simulink model "Asyn_Demodulator"  (R2014b)
settings: Solver=ode3  StartTime=0.0  StopTime=1  FixedStep=1/5000000  RelTol=1e-3
undefined symbols (not defined in the file or in its folder): dfilt, fdesignblkfcn, gcbh
libraries: dsparch4 x1
settings Model: Creator=Eitima  LastModifiedBy=Eitima
settings DataIOCC: ExternalInput=[t, SigTime]  LimitDataPoints=off  LoadExternalInput=on  TimeSaveName=tOut  OutputSaveName=SigTimeOut

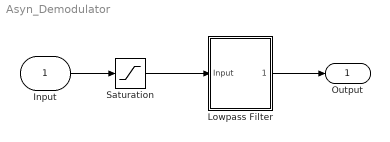
== system Asyn_Demodulator ==
  Input : Inport
  Lowpass Filter : Subsystem
  Saturation : Saturate  UpperLimit=inf  LowerLimit=0
  Output : Outport
  wires:
  Lowpass Filter/1(Output) -> Output/1
  Saturation/1 -> Lowpass Filter/1(Input)
  Input/1 -> Saturation/1

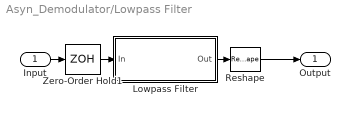
== system Asyn_Demodulator/Lowpass Filter ==
  Input : Inport
  Lowpass Filter : Subsystem  DialogController=fdesignblkfcn  InitFcn=fdesignblkfcn(gcbh, {'InitFcn'});  mask(Lowpass Filter){}
      mask help: Design a lowpass filter
      settings: CopyFcn=fdesignblkfcn(gcbh, {'CopyFcn'});
      mask Help: helpview(mapfilelocation('dsp'), 'dsplowpassfilter');
      mask Display: disp('Lowpass')
  Reshape : Reshape
  Zero-Order Hold1 : ZeroOrderHold  SampleTime=-1
  Output : Outport
  wires:
  Zero-Order Hold1/1 -> Lowpass Filter/1(In)
  Input/1 -> Zero-Order Hold1/1
  Lowpass Filter/1(Out) -> Reshape/1
  Reshape/1 -> Output/1

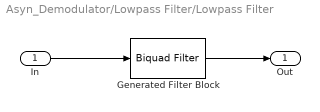
== system Asyn_Demodulator/Lowpass Filter/Lowpass Filter ==
  In : Inport
  Generated Filter Block : dsparch4/Biquad Filter  Tag=BlockMethodSubSystem  IIRFiltStruct=Direct form II  CoeffSource=Specify via dialog  BiQuadCoeffs=[1.1139495474470017e-05 2.2278990948940034e-05 1.1139495474470017e-05 1 -1.9975472496899784 0.99760587630988296;1.708449290031526e-05 3.4168985800630521e-05 1.708449290031526e-05 1 -1.99387457640288 0.99393309523238282;2.1150286544110928e-05 4.2300573088221855e-05 2.1150286544110928e-05 1 -1.9905941002634866 0.99065252281330018;2.3741131754506419e-05 4.7482263509012838e-05 2.3741131754506419e-05 1 -1.9879072271736171 0.9879655708655779;2.2148688266151217e-05 4.4297376532302434e-05 2.2148688266151217e-05 1 -1.9859774513096744 0.98603573836405833;1.4562706238119281e-05 2.9125412476238562e-05 1.4562706238119281e-05 1 -1.9849213847063547 0.98497964076591971;1.4567049256231092e-05 2.9134098512462184e-05 1.4567049256231092e-05 1 -1.9847430291087753 0.98480127993372768;1.457808673549499e-05 2.915617347098998e-05 1.457808673549499e-05 1 -1.9853349366021702 0.98539320479919512;1.4595153426943952e-05 2.9190306853887904e-05 1.4595153426943952e-05 1 -1.986839228435767 0.98689754078270897;1.4617214727563608e-05 2.9234429455127217e-05 1.4617214727563608e-05 1 -1.9891652381977778 0.98922361881148557;1.4642922502972056e-05 2.9285845005944111e-05 1.4642922502972056e-05 1 -1.9921719604380583 0.99223042929696859;8.6714112246987757e-06 1.7342822449397551e-05 8.6714112246987757e-06 1 -1.995675658652956 0.99573423034296782;6.3986527910792821e-06 1.2797305582158564e-05 6.3986527910792821e-06 1 -1.9994601364673172 0.99951881922911578;1.3142520276408514e-05 2.6285040552817028e-05 1.3142520276408514e-05 1 -1.9966044420030755 0.99666304095223146;1.8418289343954956e-05 3.6836578687909913e-05 1.8418289343954956e-05 1 -1.9930092733310447 0.99306776676450537;2.2982277427308612e-05 4.5964554854617224e-05 2.2982277427308612e-05 1 -1.9898596189140614 0.98991801990735939;2.6110938013399351e-05 5.2221876026798703e-05 2.6110938013399351e-05 1 -1.9873483912460574 0.98740671853657336;1.7614429604367743e-05 3.5228859208735487e-05 1.7614429604367743e-05 1 -1.9856280998827738 0.98568637668393688;1.4565318613601885e-05 2.9130637227203771e-05 1.4565318613601885e-05 1 -1.9848025557236171 0.98486080829563394;1.4574729484739814e-05 2.9149458969479628e-05 1.4574729484739814e-05 1 -1.9850990682844676 0.98515732955892188;1.4590372236056304e-05 2.9180744472112607e-05 1.4590372236056304e-05 1 -1.9863816706239454 0.98643996954188451;1.4611300168831942e-05 2.9222600337663884e-05 1.4611300168831942e-05 1 -1.9885136123818619 0.98857197387080598;1.4636237197718225e-05 2.9272474395436451e-05 1.4636237197718225e-05 1 -1.9913658685524318 0.99142431375310713;1.4663493412127055e-05 2.9326986824254111e-05 1.4663493412127055e-05 1 -1.9947645221736521 0.99482306712244295;0.25000264423165819 0.50000528846331638 0.25000264423165819 1 -1.9985003940838757 0.99855904867790413]  a0Flag=Warning  IC=0  ICnum=0  ICden=0  InputProcessing=Columns as channels (frame based)  denAccumFracLength=30  denProdOutputFracLength=30  secondMemoryFracLength=15  roundingMode=Floor  overflowMode=off  ScaleValues=[1.8320818000818615e-05;1;1;1;1;1;1;1;1;1;1;1;1;1;1;1;1;1;1;1;1;1;1;1;1;1]  optimizeScaleValues=off  ScaleValueMode=Specify via input port (g)  scaleValueFracLength=14  FilterSource=Specify via dialog  dfiltObjectName=dfilt.df2tsos([1 0.3 0.4],[1 0.1 0.2])
  Out : Outport
  wires:
  Generated Filter Block/1 -> Out/1
  In/1 -> Generated Filter Block/1
